simulink model "fig9_84"  (Simulink 4.00)
settings: Solver=ode45  SolverMode=SingleTasking  StartTime=0.0  StopTime=100.0  RelTol=1e-5  AbsTol=1e-6
values from neighbouring files (symbols this model uses):
  a = 1    [fig3_18.m]    (also in fig3_31.m; fig3_32a.m; fig3_32b.m = 0.5; fig3_32c.m = 0.5)
undefined symbols (not defined in the file or in its folder): b, c, d
libraries: simulink3 x1
CloseFcn:
  | ;slview('closediagram',bdroot);
settings Model: LastModifiedBy=abbas  LimitDataPoints=off  BlockReductionOpt=off

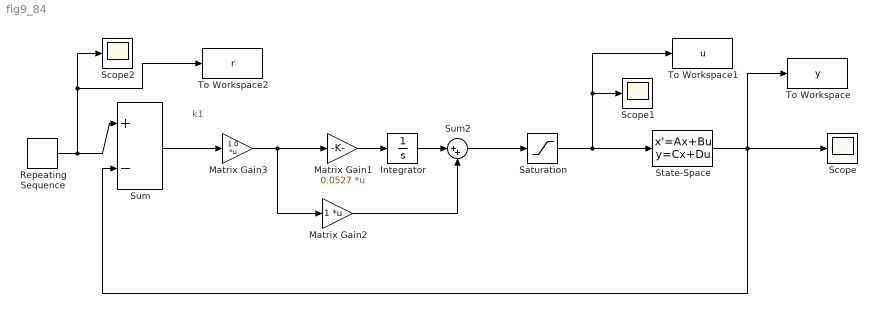
== system fig9_84 ==
  note: k1
  Integrator : Integrator  ExternalReset=none  InitialConditionSource=internal  InitialCondition=0  LimitOutput=off  UpperSaturationLimit=inf  LowerSaturationLimit=-inf  ShowSaturationPort=off  ShowStatePort=off  AbsoluteTolerance=auto
  Matrix Gain1 : Gain  Gain=0.0527  Multiplication=Matrix(K*u)  SaturateOnIntegerOverflow=on
  Matrix Gain2 : Gain  Gain=1  Multiplication=Matrix(K*u)  SaturateOnIntegerOverflow=on
  Matrix Gain3 : Gain  Gain=1.0  Multiplication=Matrix(K*u)  SaturateOnIntegerOverflow=on
  Repeating Sequence : simulink3/Sources/Repeating Sequence  rep_seq_t=[0:0.1:100]  rep_seq_y=[0:.1:25 25*ones(1,500) 0*ones(1,250)]
  Saturation : Saturate  UpperLimit=100  LowerLimit=-100  LinearizeAsGain=on
  Scope : Scope
      settings: TickLabels=on  TimeRange=100  YMin=0  YMax=100  SaveToWorkspace=off  SaveName=ScopeData  DataFormat=Array  LimitDataPoints=on  MaxDataPoints=5000
  Scope1 : Scope
      settings: TickLabels=on  TimeRange=auto  YMin=-5  YMax=5  SaveToWorkspace=off  SaveName=ScopeData  DataFormat=Array  LimitDataPoints=on  MaxDataPoints=5000
  Scope2 : Scope
      settings: TickLabels=on  TimeRange=auto  YMin=-5  YMax=5  SaveToWorkspace=off  DataFormat=Array  LimitDataPoints=on  MaxDataPoints=5000
  State-Space : StateSpace  A=a  B=b  C=c  D=d  X0=0  Realization=auto  AbsoluteTolerance=auto
  Sum : Sum  Inputs=+-  SaturateOnIntegerOverflow=on
  Sum2 : Sum  Inputs=|++  SaturateOnIntegerOverflow=on
  To Workspace : ToWorkspace  VariableName=y  SampleTime=-1  SaveFormat=Array
  To Workspace1 : ToWorkspace  VariableName=u  SampleTime=-1  SaveFormat=Array
  To Workspace2 : ToWorkspace  VariableName=r  SampleTime=-1  SaveFormat=Array
  wires:
  Matrix Gain1/1 -> Integrator/1
  State-Space/1 -> Scope/1, Sum/2, To Workspace/1
  Matrix Gain2/1 -> Sum2/2
  Integrator/1 -> Sum2/1
  Sum2/1 -> Saturation/1
  Saturation/1 -> State-Space/1, Scope1/1, To Workspace1/1
  Sum/1 -> Matrix Gain3/1
  Matrix Gain3/1 -> Matrix Gain1/1, Matrix Gain2/1
  Repeating Sequence/1 -> Sum/1, Scope2/1, To Workspace2/1
